simulink model "Test_FourMotor_PID_Ave"  (R2025a)
settings: Solver=ode4  StartTime=0.0  StopTime=2  FixedStep=60e-6  RelTol=1e-3
values from neighbouring files (symbols this model uses):
  Ts = 2e-6    (= 2e-06)    [param.m]
  ts_vec = 60e-6    (= 6e-05)    [param.m]
undefined symbols (not defined in the file or in its folder): DiscIntNeverNeededParam, gcbh, HEV_Param, Limit, magnitude, motorctrl, RPM, sps_rtmsupport
libraries: fl_lib x39, spsCurrentMeasurementLib x26, spsIdealSwitchLib x24, nesl_utility x22, spsVoltageMeasurementLib x21, simulink_extras x13, spsControlledCurrentSourceLib x12, spsControlledVoltageSourceLib x9, slpidlib x7, simulink x6, Uav_Electrical_lib x5, spsSeriesRLCBranchLib x4
(part 4 of 5)

== system Test_FourMotor_PID_Ave/Detailed/Synchronous Motor & Drive1/Three-phase Inverter/Id computation ==
  m : Inport
  Vdc : Inport  Port=2
  Demux : Subsystem
  Demux1 : Subsystem
  Gain : Gain  Gain=Ron
  Math Function : Math  Operator=magnitude^2  SignedPower=on
  Math Function1 : Math  Operator=magnitude^2  SignedPower=on
  Math Function2 : Math  Operator=magnitude^2  SignedPower=on
  Product1 : Product  Inputs=*/  SaturateOnIntegerOverflow=on  OutDataTypeStr=Inherit: Same as first input
  Sum1 : Sum  Inputs=+++  SaturateOnIntegerOverflow=on
  Sum2 : Sum  Inputs=|++  SaturateOnIntegerOverflow=on
  Sum3 : Sum  SaturateOnIntegerOverflow=on
  Unit Delay1 : UnitDelay  SampleTime=Ts  HasFrameUpgradeWarning=on
  Unit Delay4 : UnitDelay  InitialCondition=1  SampleTime=Ts  HasFrameUpgradeWarning=on
  Vac x Ia : Product  SaturateOnIntegerOverflow=on  OutDataTypeStr=Inherit: Same as first input
  Vbc x Ib : Product  SaturateOnIntegerOverflow=on  OutDataTypeStr=Inherit: Same as first input
  Zero avoider : Saturate  UpperLimit=inf  LowerLimit=1
  Id : Outport  VectorParamsAs1DForOutWhenUnconnected=off
  wires:
  Sum2/1 -> Unit Delay1/1
  Sum3/1 -> Sum2/1
  Sum1/1 -> Gain/1
  Math Function2/1 -> Sum1/3
  Math Function/1 -> Sum1/1
  Math Function1/1 -> Sum1/2
  Demux1/3(Ic) -> Math Function2/1
  Demux1/2(Ib) -> Math Function1/1
  Demux1/1(Ia) -> Math Function/1
  Unit Delay4/1 -> Zero avoider/1
  Unit Delay1/1 -> Product1/1
  m/1 -> Demux1/1(m), Demux/1(m)
  Vac x Ia/1 -> Sum3/1
  Vbc x Ib/1 -> Sum3/2
  Vdc/1 -> Unit Delay4/1
  Demux/1(Vac) -> Vac x Ia/1
  Demux/2(Ia) -> Vac x Ia/2
  Demux/4(Ib) -> Vbc x Ib/2
  Demux/3(Vbc) -> Vbc x Ib/1
  Gain/1 -> Sum2/2
  Product1/1 -> Id/1
  Zero avoider/1 -> Product1/2

== system Test_FourMotor_PID_Ave/Detailed/Synchronous Motor & Drive1/Three-phase Inverter/Limit detection ==
  note: Limit = 1 saturation mode (voltage mode)
      | Limit = 0 normal mode (current mode)
  note: Low pass filter
  note: Low pass filter
  Vcc : Inport
  ctrl : Inport  Port=2
  Bus Selector1 : BusSelector  OutputSignals=m.Stator current is_d (A),m.Stator current is_q (A),m.Rotor speed wm (rad/s)  OutputAsBus=on
  Discrete Transfer Fcn1 : DiscreteTransferFcn  Numerator=[1-exp(-Ts*Fcs*2*pi)]  Denominator=[1 -exp(-Ts*Fcs*2*pi)]  SampleTime=Ts
  Discrete Transfer Fcn3 : DiscreteTransferFcn  Numerator=[1-exp(-Ts*Fcs*2*pi)]  Denominator=[1 -exp(-Ts*Fcs*2*pi)]  SampleTime=Ts
  Gain1 : Gain  Gain=0.9  SaturateOnIntegerOverflow=on  OutDataTypeStr=Inherit: Same as input  ParamDataTypeStr=Inherit: Same as input
  "Internal Vcc " : Fcn  Expr=pi/2*sqrt((Resistance*u(1)-Lq*p*u(3)*u(2))^2+(Resistance*u(2)+Ld*p*u(3)*u(1)+Flux*p*u(3))^2)
  Relational Operator : RelationalOperator  Operator=>  OutDataTypeStr=boolean  InputSameDT=off
  Relational Operator2 : RelationalOperator  Operator=<  OutDataTypeStr=boolean  InputSameDT=off
  S-R Flip-Flop : simulink_extras/Flip Flops/S-R Flip-Flop  initial_condition=0
  Terminator : Terminator
  Limit : Outport  VectorParamsAs1DForOutWhenUnconnected=off
  wires:
  Vcc/1 -> Discrete Transfer Fcn3/1
  Relational Operator/1 -> S-R Flip-Flop/1
  Relational Operator2/1 -> S-R Flip-Flop/2
  S-R Flip-Flop/1 -> Limit/1
  ctrl/1 -> Bus Selector1/1
  Bus Selector1/1 -> "Internal Vcc "/1
  "Internal Vcc "/1 -> Discrete Transfer Fcn1/1
  Discrete Transfer Fcn1/1 -> Relational Operator/1, Relational Operator2/1
  Gain1/1 -> Relational Operator2/2
  Discrete Transfer Fcn3/1 -> Gain1/1, Relational Operator/2
  S-R Flip-Flop/2 -> Terminator/1

== system Test_FourMotor_PID_Ave/Detailed/Synchronous Motor & Drive1/Three-phase Inverter/Output Resistance correction ==
  note: Vabc
  ctrl : Inport
  1/R : Gain  Gain=1/(100*Resistance)  SaturateOnIntegerOverflow=on  OutDataTypeStr=Inherit: Same as input  ParamDataTypeStr=Inherit: Same as input
  Bus Selector1 : BusSelector  OutputSignals=m.Stator voltage Vs_d (V),m.Stator voltage Vs_q (V),m.Rotor angle thetam (rad)
  Constant : Constant  Value=0
  Discrete Transfer Fcn1 : DiscreteTransferFcn  Numerator=[1-exp(-Ts/.001)]  Denominator=[1 -exp(-Ts/.001)]  SampleTime=Ts
  Discrete Transfer Fcn2 : DiscreteTransferFcn  Numerator=[1-exp(-Ts/.001)]  Denominator=[1 -exp(-Ts/.001)]  SampleTime=Ts
  Fcn : Fcn  Expr=sin(u)
  Fcn1 : Fcn  Expr=cos(u)
  Mux4 : Mux  Inputs=3
  Mux5 : Mux  Inputs=2
  dq0_to_abc Transformation : powerlib_extras/Measurements/dq0_to_abc Transformation
  poles : Gain  Gain=p  SaturateOnIntegerOverflow=on  OutDataTypeStr=Inherit: Same as input  ParamDataTypeStr=Inherit: Same as input
  "Iabc_r " : Outport  VectorParamsAs1DForOutWhenUnconnected=off
  wires:
  1/R/1 -> "Iabc_r "/1
  Bus Selector1/2 -> Discrete Transfer Fcn2/1  "<Stator voltage Vs_q (V)>"
  Bus Selector1/1 -> Discrete Transfer Fcn1/1  "<Stator voltage Vs_d (V)>"
  ctrl/1 -> Bus Selector1/1
  Mux4/1 -> dq0_to_abc Transformation/1
  Fcn/1 -> Mux5/1
  Fcn1/1 -> Mux5/2
  Mux5/1 -> dq0_to_abc Transformation/2
  Constant/1 -> Mux4/3
  dq0_to_abc Transformation/1 -> 1/R/1
  Discrete Transfer Fcn2/1 -> Mux4/2
  Discrete Transfer Fcn1/1 -> Mux4/1
  Bus Selector1/3 -> poles/1  "<Rotor angle thetam (rad)>"
  poles/1 -> Fcn/1, Fcn1/1

== system Test_FourMotor_PID_Ave/Detailed/Synchronous Motor & Drive1/VECT Controller/Current Regulator1 ==
  Iabc* : Inport
  Iabc : Inport  Port=2
  BusCreator : BusCreator  Inputs=6
  Data Type Conversion{,1..5} (6 alike) : DataTypeConversion
  Demux1 : Demux  Outputs=3
      settings: DisplayOption=none
  Demux2 : Demux  Outputs=3
      settings: DisplayOption=none
  Logical Operator : Logic  Operator=NOT
  Logical Operator1 : Logic  Operator=NOT
  Logical Operator2 : Logic  Operator=NOT
  Relay : Relay  OnSwitchValue=h/2  OffSwitchValue=-h/2
  Relay1 : Relay  OnSwitchValue=h/2  OffSwitchValue=-h/2
  Relay2 : Relay  OnSwitchValue=h/2  OffSwitchValue=-h/2
  Sum : Sum  Inputs=-+  InputSameDT=on  SaturateOnIntegerOverflow=on  OutDataTypeStr=Inherit: Same as first input
  Sum1 : Sum  Inputs=-+  InputSameDT=on  SaturateOnIntegerOverflow=on  OutDataTypeStr=Inherit: Same as first input
  Sum2 : Sum  Inputs=-+  InputSameDT=on  SaturateOnIntegerOverflow=on  OutDataTypeStr=Inherit: Same as first input
  Pulses : Outport  InitialOutput=0  VectorParamsAs1DForOutWhenUnconnected=off
  wires:
  Data Type Conversion5/1 -> BusCreator/6
  Data Type Conversion4/1 -> Logical Operator2/1
  Data Type Conversion3/1 -> BusCreator/4
  Data Type Conversion2/1 -> Logical Operator1/1
  Data Type Conversion1/1 -> BusCreator/2
  Data Type Conversion/1 -> Logical Operator/1
  Sum/1 -> Relay/1
  Sum1/1 -> Relay1/1
  Demux1/1 -> Sum/1
  Demux1/2 -> Sum1/1
  BusCreator/1 -> Pulses/1
  Iabc/1 -> Demux1/1
  Sum2/1 -> Relay2/1
  Demux1/3 -> Sum2/1
  Demux2/3 -> Sum2/2
  Demux2/2 -> Sum1/2
  Demux2/1 -> Sum/2
  Iabc*/1 -> Demux2/1
  Relay/1 -> Data Type Conversion/1, BusCreator/1
  Relay1/1 -> Data Type Conversion2/1, BusCreator/3
  Relay2/1 -> Data Type Conversion4/1, BusCreator/5
  Logical Operator/1 -> Data Type Conversion1/1
  Logical Operator1/1 -> Data Type Conversion3/1
  Logical Operator2/1 -> Data Type Conversion5/1

== system Test_FourMotor_PID_Ave/Detailed/Synchronous Motor & Drive1/VECT Controller/DQ-ABC ==
  "Iq* " : Inport
  "Id* " : Inport  Port=2
  Teta : Inport  Port=3
  Fcn : Fcn  Expr=sin(u)
  Fcn1 : Fcn  Expr=cos(u)
  Gain2 : Gain  SaturateOnIntegerOverflow=on  OutDataTypeStr=Inherit: Same as input  ParamDataTypeStr=Inherit: Same as input
  Gain3 : Gain  SaturateOnIntegerOverflow=on  OutDataTypeStr=Inherit: Same as input  ParamDataTypeStr=Inherit: Same as input
  Gain4 : Gain  SaturateOnIntegerOverflow=on  OutDataTypeStr=Inherit: Same as input  ParamDataTypeStr=Inherit: Same as input
  Mux : Mux
  Mux2 : Mux  Inputs=3
  ia : Fcn  Expr=-u[3]*u[2] + u[4]*u[1]
  ib : Fcn  Expr=(-u[1]+1.7320508*u[2])*u[4]*0.5+(u[2]+1.7320508*u[1])*u[3]*0.5
  ic : Sum  Inputs=--  InputSameDT=on  SaturateOnIntegerOverflow=on  OutDataTypeStr=Inherit: Same as first input
  Iabc* : Outport  InitialOutput=0  VectorParamsAs1DForOutWhenUnconnected=off
  wires:
  ib/1 -> ic/1, Gain3/1
  ia/1 -> ic/2, Gain2/1
  Gain2/1 -> Mux2/1
  Gain4/1 -> Mux2/3
  ic/1 -> Gain4/1
  Gain3/1 -> Mux2/2
  "Iq* "/1 -> Mux/4
  "Id* "/1 -> Mux/3
  Teta/1 -> Fcn/1, Fcn1/1
  Mux/1 -> ia/1, ib/1
  Mux2/1 -> Iabc*/1
  Fcn1/1 -> Mux/1
  Fcn/1 -> Mux/2

== system Test_FourMotor_PID_Ave/Detailed/Synchronous Motor & Drive2/Three-phase Inverter/Activation Switches ==
  gate : Inport
  Ideal Switch1 : spsIdealSwitchLib/Ideal Switch  Ron=2*Ron  Lon=0  IC=1  Rs=1e6  Cs=inf  Measurements=off
  Ideal Switch2 : spsIdealSwitchLib/Ideal Switch  Ron=2*Ron  Lon=0  IC=1  Rs=1e6  Cs=inf  Measurements=off
  Ideal Switch3 : spsIdealSwitchLib/Ideal Switch  Ron=2*Ron  Lon=0  IC=1  Rs=1e6  Cs=inf  Measurements=off
  Ideal Switch4 : spsIdealSwitchLib/Ideal Switch  Ron=2*Ron  Lon=0  IC=0  Rs=1e6  Cs=inf  Measurements=off
  Ideal Switch5 : spsIdealSwitchLib/Ideal Switch  Ron=2*Ron  Lon=0  IC=0  Rs=1e6  Cs=inf  Measurements=off
  Ideal Switch6 : spsIdealSwitchLib/Ideal Switch  Ron=2*Ron  Lon=0  IC=0  Rs=1e6  Cs=inf  Measurements=off
  Logical Operator : Logic  Operator=NOT  AllPortsSameDT=off  OutDataTypeStr=boolean
  A1 : PMIOPort  Side=Left
  a : PMIOPort  Port=2  Side=Right
  B1 : PMIOPort  Port=3  Side=Left
  b : PMIOPort  Port=4  Side=Right
  C1 : PMIOPort  Port=5  Side=Left
  c : PMIOPort  Port=6  Side=Right
  A2 : PMIOPort  Port=7  Side=Left
  B2 : PMIOPort  Port=8  Side=Left
  C2 : PMIOPort  Port=9  Side=Left
  wires:
  gate/1 -> Ideal Switch1/1, Ideal Switch2/1, Ideal Switch3/1, Logical Operator/1
  Logical Operator/1 -> Ideal Switch4/1, Ideal Switch5/1, Ideal Switch6/1
  connections:
  A1/RConn1 -- Ideal Switch1/LConn1
  Ideal Switch1/RConn1 -- a/RConn1 -- Ideal Switch4/RConn1
  B1/RConn1 -- Ideal Switch2/LConn1
  Ideal Switch2/RConn1 -- Ideal Switch5/RConn1 -- b/RConn1
  C1/RConn1 -- Ideal Switch3/LConn1
  Ideal Switch3/RConn1 -- Ideal Switch6/RConn1 -- c/RConn1
  A2/RConn1 -- Ideal Switch4/LConn1
  B2/RConn1 -- Ideal Switch5/LConn1
  C2/RConn1 -- Ideal Switch6/LConn1

== system Test_FourMotor_PID_Ave/Detailed/Synchronous Motor & Drive2/Three-phase Inverter/Id computation ==
  m : Inport
  Vdc : Inport  Port=2
  Demux : Subsystem
  Demux1 : Subsystem
  Gain : Gain  Gain=Ron
  Math Function : Math  Operator=magnitude^2  SignedPower=on
  Math Function1 : Math  Operator=magnitude^2  SignedPower=on
  Math Function2 : Math  Operator=magnitude^2  SignedPower=on
  Product1 : Product  Inputs=*/  SaturateOnIntegerOverflow=on  OutDataTypeStr=Inherit: Same as first input
  Sum1 : Sum  Inputs=+++  SaturateOnIntegerOverflow=on
  Sum2 : Sum  Inputs=|++  SaturateOnIntegerOverflow=on
  Sum3 : Sum  SaturateOnIntegerOverflow=on
  Unit Delay1 : UnitDelay  SampleTime=Ts  HasFrameUpgradeWarning=on
  Unit Delay4 : UnitDelay  InitialCondition=1  SampleTime=Ts  HasFrameUpgradeWarning=on
  Vac x Ia : Product  SaturateOnIntegerOverflow=on  OutDataTypeStr=Inherit: Same as first input
  Vbc x Ib : Product  SaturateOnIntegerOverflow=on  OutDataTypeStr=Inherit: Same as first input
  Zero avoider : Saturate  UpperLimit=inf  LowerLimit=1
  Id : Outport  VectorParamsAs1DForOutWhenUnconnected=off
  wires:
  Sum2/1 -> Unit Delay1/1
  Sum3/1 -> Sum2/1
  Sum1/1 -> Gain/1
  Math Function2/1 -> Sum1/3
  Math Function/1 -> Sum1/1
  Math Function1/1 -> Sum1/2
  Demux1/3(Ic) -> Math Function2/1
  Demux1/2(Ib) -> Math Function1/1
  Demux1/1(Ia) -> Math Function/1
  Unit Delay4/1 -> Zero avoider/1
  Unit Delay1/1 -> Product1/1
  m/1 -> Demux1/1(m), Demux/1(m)
  Vac x Ia/1 -> Sum3/1
  Vbc x Ib/1 -> Sum3/2
  Vdc/1 -> Unit Delay4/1
  Demux/1(Vac) -> Vac x Ia/1
  Demux/2(Ia) -> Vac x Ia/2
  Demux/4(Ib) -> Vbc x Ib/2
  Demux/3(Vbc) -> Vbc x Ib/1
  Gain/1 -> Sum2/2
  Product1/1 -> Id/1
  Zero avoider/1 -> Product1/2

== system Test_FourMotor_PID_Ave/Detailed/Synchronous Motor & Drive2/Three-phase Inverter/Limit detection ==
  note: Limit = 1 saturation mode (voltage mode)
      | Limit = 0 normal mode (current mode)
  note: Low pass filter
  note: Low pass filter
  Vcc : Inport
  ctrl : Inport  Port=2
  Bus Selector1 : BusSelector  OutputSignals=m.Stator current is_d (A),m.Stator current is_q (A),m.Rotor speed wm (rad/s)  OutputAsBus=on
  Discrete Transfer Fcn1 : DiscreteTransferFcn  Numerator=[1-exp(-Ts*Fcs*2*pi)]  Denominator=[1 -exp(-Ts*Fcs*2*pi)]  SampleTime=Ts
  Discrete Transfer Fcn3 : DiscreteTransferFcn  Numerator=[1-exp(-Ts*Fcs*2*pi)]  Denominator=[1 -exp(-Ts*Fcs*2*pi)]  SampleTime=Ts
  Gain1 : Gain  Gain=0.9  SaturateOnIntegerOverflow=on  OutDataTypeStr=Inherit: Same as input  ParamDataTypeStr=Inherit: Same as input
  "Internal Vcc " : Fcn  Expr=pi/2*sqrt((Resistance*u(1)-Lq*p*u(3)*u(2))^2+(Resistance*u(2)+Ld*p*u(3)*u(1)+Flux*p*u(3))^2)
  Relational Operator : RelationalOperator  Operator=>  OutDataTypeStr=boolean  InputSameDT=off
  Relational Operator2 : RelationalOperator  Operator=<  OutDataTypeStr=boolean  InputSameDT=off
  S-R Flip-Flop : simulink_extras/Flip Flops/S-R Flip-Flop  initial_condition=0
  Terminator : Terminator
  Limit : Outport  VectorParamsAs1DForOutWhenUnconnected=off
  wires:
  Vcc/1 -> Discrete Transfer Fcn3/1
  Relational Operator/1 -> S-R Flip-Flop/1
  Relational Operator2/1 -> S-R Flip-Flop/2
  S-R Flip-Flop/1 -> Limit/1
  ctrl/1 -> Bus Selector1/1
  Bus Selector1/1 -> "Internal Vcc "/1
  "Internal Vcc "/1 -> Discrete Transfer Fcn1/1
  Discrete Transfer Fcn1/1 -> Relational Operator/1, Relational Operator2/1
  Gain1/1 -> Relational Operator2/2
  Discrete Transfer Fcn3/1 -> Gain1/1, Relational Operator/2
  S-R Flip-Flop/2 -> Terminator/1

== system Test_FourMotor_PID_Ave/Detailed/Synchronous Motor & Drive2/Three-phase Inverter/Output Resistance correction ==
  note: Vabc
  ctrl : Inport
  1/R : Gain  Gain=1/(100*Resistance)  SaturateOnIntegerOverflow=on  OutDataTypeStr=Inherit: Same as input  ParamDataTypeStr=Inherit: Same as input
  Bus Selector1 : BusSelector  OutputSignals=m.Stator voltage Vs_d (V),m.Stator voltage Vs_q (V),m.Rotor angle thetam (rad)
  Constant : Constant  Value=0
  Discrete Transfer Fcn1 : DiscreteTransferFcn  Numerator=[1-exp(-Ts/.001)]  Denominator=[1 -exp(-Ts/.001)]  SampleTime=Ts
  Discrete Transfer Fcn2 : DiscreteTransferFcn  Numerator=[1-exp(-Ts/.001)]  Denominator=[1 -exp(-Ts/.001)]  SampleTime=Ts
  Fcn : Fcn  Expr=sin(u)
  Fcn1 : Fcn  Expr=cos(u)
  Mux4 : Mux  Inputs=3
  Mux5 : Mux  Inputs=2
  dq0_to_abc Transformation : powerlib_extras/Measurements/dq0_to_abc Transformation
  poles : Gain  Gain=p  SaturateOnIntegerOverflow=on  OutDataTypeStr=Inherit: Same as input  ParamDataTypeStr=Inherit: Same as input
  "Iabc_r " : Outport  VectorParamsAs1DForOutWhenUnconnected=off
  wires:
  1/R/1 -> "Iabc_r "/1
  Bus Selector1/2 -> Discrete Transfer Fcn2/1  "<Stator voltage Vs_q (V)>"
  Bus Selector1/1 -> Discrete Transfer Fcn1/1  "<Stator voltage Vs_d (V)>"
  ctrl/1 -> Bus Selector1/1
  Mux4/1 -> dq0_to_abc Transformation/1
  Fcn/1 -> Mux5/1
  Fcn1/1 -> Mux5/2
  Mux5/1 -> dq0_to_abc Transformation/2
  Constant/1 -> Mux4/3
  dq0_to_abc Transformation/1 -> 1/R/1
  Discrete Transfer Fcn2/1 -> Mux4/2
  Discrete Transfer Fcn1/1 -> Mux4/1
  Bus Selector1/3 -> poles/1  "<Rotor angle thetam (rad)>"
  poles/1 -> Fcn/1, Fcn1/1

== system Test_FourMotor_PID_Ave/Detailed/Synchronous Motor & Drive2/VECT controller/Current Regulator ==
  Iabc* : Inport
  Iabc : Inport  Port=2
  Demux1 : Demux  Outputs=3
      settings: DisplayOption=none
  Demux2 : Demux  Outputs=3
      settings: DisplayOption=none
  Mux1 : Mux  Inputs=2
  Relay : Relay  OnSwitchValue=0  OffSwitchValue=0
  Relay1 : Relay  OnSwitchValue=0  OffSwitchValue=0
  Relay2 : Relay  OnSwitchValue=0  OffSwitchValue=0
  Sum : Sum  Inputs=-+  InputSameDT=on  SaturateOnIntegerOverflow=on  OutDataTypeStr=Inherit: Same as first input
  Sum1 : Sum  Inputs=-+  InputSameDT=on  SaturateOnIntegerOverflow=on  OutDataTypeStr=Inherit: Same as first input
  Sum2 : Sum  Inputs=-+  InputSameDT=on  SaturateOnIntegerOverflow=on  OutDataTypeStr=Inherit: Same as first input
  Sum3 : Sum  Inputs=+-
  Sum4 : Sum  Inputs=+-
  Pulses : Outport  InitialOutput=0  VectorParamsAs1DForOutWhenUnconnected=off
  wires:
  Sum/1 -> Relay/1
  Sum1/1 -> Relay1/1
  Demux1/1 -> Sum/1
  Demux1/2 -> Sum1/1
  Mux1/1 -> Pulses/1
  Iabc/1 -> Demux1/1
  Sum2/1 -> Relay2/1
  Demux1/3 -> Sum2/1
  Demux2/3 -> Sum2/2
  Demux2/2 -> Sum1/2
  Demux2/1 -> Sum/2
  Iabc*/1 -> Demux2/1
  Relay/1 -> Sum3/1
  Relay1/1 -> Sum3/2, Sum4/1
  Relay2/1 -> Sum4/2
  Sum3/1 -> Mux1/1
  Sum4/1 -> Mux1/2

== system Test_FourMotor_PID_Ave/Detailed/Synchronous Motor & Drive2/VECT controller/DQ-ABC ==
  "Iq* " : Inport
  "Id* " : Inport  Port=2
  Teta : Inport  Port=3
  Fcn : Fcn  Expr=sin(u)
  Fcn1 : Fcn  Expr=cos(u)
  Gain2 : Gain  SaturateOnIntegerOverflow=on  OutDataTypeStr=Inherit: Same as input  ParamDataTypeStr=Inherit: Same as input
  Gain3 : Gain  SaturateOnIntegerOverflow=on  OutDataTypeStr=Inherit: Same as input  ParamDataTypeStr=Inherit: Same as input
  Gain4 : Gain  SaturateOnIntegerOverflow=on  OutDataTypeStr=Inherit: Same as input  ParamDataTypeStr=Inherit: Same as input
  Mux : Mux
  Mux2 : Mux  Inputs=3
  ia : Fcn  Expr=-u[3]*u[2] + u[4]*u[1]
  ib : Fcn  Expr=(-u[1]+1.7320508*u[2])*u[4]*0.5+(u[2]+1.7320508*u[1])*u[3]*0.5
  ic : Sum  Inputs=--  InputSameDT=on  SaturateOnIntegerOverflow=on  OutDataTypeStr=Inherit: Same as first input
  Iabc* : Outport  InitialOutput=0  VectorParamsAs1DForOutWhenUnconnected=off
  wires:
  Fcn/1 -> Mux/2
  Fcn1/1 -> Mux/1
  Mux2/1 -> Iabc*/1
  Mux/1 -> ib/1, ia/1
  Teta/1 -> Fcn1/1, Fcn/1
  "Id* "/1 -> Mux/3
  "Iq* "/1 -> Mux/4
  Gain3/1 -> Mux2/2
  ic/1 -> Gain4/1
  Gain4/1 -> Mux2/3
  Gain2/1 -> Mux2/1
  ia/1 -> Gain2/1, ic/2
  ib/1 -> Gain3/1, ic/1

== system Test_FourMotor_PID_Ave/Detailed/Synchronous Motor & Drive2/VECT controller/Zero crossing detector ==
  En : Inport
  Iabc* : Inport  Port=2
  D Latch : simulink_extras/Flip Flops/D Latch
  D Latch1 : simulink_extras/Flip Flops/D Latch
  D Latch2 : simulink_extras/Flip Flops/D Latch
  Data Type Conversion : DataTypeConversion  SaturateOnIntegerOverflow=off  RndMeth=Floor
  Data Type Conversion2 : DataTypeConversion  SaturateOnIntegerOverflow=off  RndMeth=Floor
  Demux : Demux  Outputs=3
  Hit Crossing : HitCross
  Mux : Mux  Inputs=3
  Terminator : Terminator
  Terminator1 : Terminator
  Terminator2 : Terminator
  Enable : Outport  VectorParamsAs1DForOutWhenUnconnected=off
  wires:
  Data Type Conversion/1 -> D Latch/1, D Latch1/1, D Latch2/1
  Hit Crossing/1 -> Demux/1
  Demux/2 -> D Latch1/2
  Demux/3 -> D Latch2/2
  D Latch/1 -> Mux/1
  D Latch1/1 -> Mux/2
  D Latch2/1 -> Mux/3
  Mux/1 -> Data Type Conversion2/1
  Demux/1 -> D Latch/2
  En/1 -> Data Type Conversion/1
  Iabc*/1 -> Hit Crossing/1
  Data Type Conversion2/1 -> Enable/1
  D Latch/2 -> Terminator/1
  D Latch1/2 -> Terminator1/1
  D Latch2/2 -> Terminator2/1

== system Test_FourMotor_PID_Ave/Detailed/Synchronous Motor & Drive3/Three-phase Inverter/Activation Switches ==
  gate : Inport
  Ideal Switch1 : spsIdealSwitchLib/Ideal Switch  Ron=2*Ron  Lon=0  IC=1  Rs=1e6  Cs=inf  Measurements=off
  Ideal Switch2 : spsIdealSwitchLib/Ideal Switch  Ron=2*Ron  Lon=0  IC=1  Rs=1e6  Cs=inf  Measurements=off
  Ideal Switch3 : spsIdealSwitchLib/Ideal Switch  Ron=2*Ron  Lon=0  IC=1  Rs=1e6  Cs=inf  Measurements=off
  Ideal Switch4 : spsIdealSwitchLib/Ideal Switch  Ron=2*Ron  Lon=0  IC=0  Rs=1e6  Cs=inf  Measurements=off
  Ideal Switch5 : spsIdealSwitchLib/Ideal Switch  Ron=2*Ron  Lon=0  IC=0  Rs=1e6  Cs=inf  Measurements=off
  Ideal Switch6 : spsIdealSwitchLib/Ideal Switch  Ron=2*Ron  Lon=0  IC=0  Rs=1e6  Cs=inf  Measurements=off
  Logical Operator : Logic  Operator=NOT  AllPortsSameDT=off  OutDataTypeStr=boolean
  A1 : PMIOPort  Side=Left
  a : PMIOPort  Port=2  Side=Right
  B1 : PMIOPort  Port=3  Side=Left
  b : PMIOPort  Port=4  Side=Right
  C1 : PMIOPort  Port=5  Side=Left
  c : PMIOPort  Port=6  Side=Right
  A2 : PMIOPort  Port=7  Side=Left
  B2 : PMIOPort  Port=8  Side=Left
  C2 : PMIOPort  Port=9  Side=Left
  wires:
  gate/1 -> Ideal Switch1/1, Ideal Switch2/1, Ideal Switch3/1, Logical Operator/1
  Logical Operator/1 -> Ideal Switch4/1, Ideal Switch5/1, Ideal Switch6/1
  connections:
  A1/RConn1 -- Ideal Switch1/LConn1
  Ideal Switch1/RConn1 -- a/RConn1 -- Ideal Switch4/RConn1
  B1/RConn1 -- Ideal Switch2/LConn1
  Ideal Switch2/RConn1 -- Ideal Switch5/RConn1 -- b/RConn1
  C1/RConn1 -- Ideal Switch3/LConn1
  Ideal Switch3/RConn1 -- Ideal Switch6/RConn1 -- c/RConn1
  A2/RConn1 -- Ideal Switch4/LConn1
  B2/RConn1 -- Ideal Switch5/LConn1
  C2/RConn1 -- Ideal Switch6/LConn1

== system Test_FourMotor_PID_Ave/Detailed/Synchronous Motor & Drive3/Three-phase Inverter/Id computation ==
  m : Inport
  Vdc : Inport  Port=2
  Demux : Subsystem
  Demux1 : Subsystem
  Gain : Gain  Gain=Ron
  Math Function : Math  Operator=magnitude^2  SignedPower=on
  Math Function1 : Math  Operator=magnitude^2  SignedPower=on
  Math Function2 : Math  Operator=magnitude^2  SignedPower=on
  Product1 : Product  Inputs=*/  SaturateOnIntegerOverflow=on  OutDataTypeStr=Inherit: Same as first input
  Sum1 : Sum  Inputs=+++  SaturateOnIntegerOverflow=on
  Sum2 : Sum  Inputs=|++  SaturateOnIntegerOverflow=on
  Sum3 : Sum  SaturateOnIntegerOverflow=on
  Unit Delay1 : UnitDelay  SampleTime=Ts  HasFrameUpgradeWarning=on
  Unit Delay4 : UnitDelay  InitialCondition=1  SampleTime=Ts  HasFrameUpgradeWarning=on
  Vac x Ia : Product  SaturateOnIntegerOverflow=on  OutDataTypeStr=Inherit: Same as first input
  Vbc x Ib : Product  SaturateOnIntegerOverflow=on  OutDataTypeStr=Inherit: Same as first input
  Zero avoider : Saturate  UpperLimit=inf  LowerLimit=1
  Id : Outport  VectorParamsAs1DForOutWhenUnconnected=off
  wires:
  Sum2/1 -> Unit Delay1/1
  Sum3/1 -> Sum2/1
  Sum1/1 -> Gain/1
  Math Function2/1 -> Sum1/3
  Math Function/1 -> Sum1/1
  Math Function1/1 -> Sum1/2
  Demux1/3(Ic) -> Math Function2/1
  Demux1/2(Ib) -> Math Function1/1
  Demux1/1(Ia) -> Math Function/1
  Unit Delay4/1 -> Zero avoider/1
  Unit Delay1/1 -> Product1/1
  m/1 -> Demux1/1(m), Demux/1(m)
  Vac x Ia/1 -> Sum3/1
  Vbc x Ib/1 -> Sum3/2
  Vdc/1 -> Unit Delay4/1
  Demux/1(Vac) -> Vac x Ia/1
  Demux/2(Ia) -> Vac x Ia/2
  Demux/4(Ib) -> Vbc x Ib/2
  Demux/3(Vbc) -> Vbc x Ib/1
  Gain/1 -> Sum2/2
  Product1/1 -> Id/1
  Zero avoider/1 -> Product1/2

== system Test_FourMotor_PID_Ave/Detailed/Synchronous Motor & Drive3/Three-phase Inverter/Limit detection ==
  note: Limit = 1 saturation mode (voltage mode)
      | Limit = 0 normal mode (current mode)
  note: Low pass filter
  note: Low pass filter
  Vcc : Inport
  ctrl : Inport  Port=2
  Bus Selector1 : BusSelector  OutputSignals=m.Stator current is_d (A),m.Stator current is_q (A),m.Rotor speed wm (rad/s)  OutputAsBus=on
  Discrete Transfer Fcn1 : DiscreteTransferFcn  Numerator=[1-exp(-Ts*Fcs*2*pi)]  Denominator=[1 -exp(-Ts*Fcs*2*pi)]  SampleTime=Ts
  Discrete Transfer Fcn3 : DiscreteTransferFcn  Numerator=[1-exp(-Ts*Fcs*2*pi)]  Denominator=[1 -exp(-Ts*Fcs*2*pi)]  SampleTime=Ts
  Gain1 : Gain  Gain=0.9  SaturateOnIntegerOverflow=on  OutDataTypeStr=Inherit: Same as input  ParamDataTypeStr=Inherit: Same as input
  "Internal Vcc " : Fcn  Expr=pi/2*sqrt((Resistance*u(1)-Lq*p*u(3)*u(2))^2+(Resistance*u(2)+Ld*p*u(3)*u(1)+Flux*p*u(3))^2)
  Relational Operator : RelationalOperator  Operator=>  OutDataTypeStr=boolean  InputSameDT=off
  Relational Operator2 : RelationalOperator  Operator=<  OutDataTypeStr=boolean  InputSameDT=off
  S-R Flip-Flop : simulink_extras/Flip Flops/S-R Flip-Flop  initial_condition=0
  Terminator : Terminator
  Limit : Outport  VectorParamsAs1DForOutWhenUnconnected=off
  wires:
  Vcc/1 -> Discrete Transfer Fcn3/1
  Relational Operator/1 -> S-R Flip-Flop/1
  Relational Operator2/1 -> S-R Flip-Flop/2
  S-R Flip-Flop/1 -> Limit/1
  ctrl/1 -> Bus Selector1/1
  Bus Selector1/1 -> "Internal Vcc "/1
  "Internal Vcc "/1 -> Discrete Transfer Fcn1/1
  Discrete Transfer Fcn1/1 -> Relational Operator/1, Relational Operator2/1
  Gain1/1 -> Relational Operator2/2
  Discrete Transfer Fcn3/1 -> Gain1/1, Relational Operator/2
  S-R Flip-Flop/2 -> Terminator/1

== system Test_FourMotor_PID_Ave/Detailed/Synchronous Motor & Drive3/Three-phase Inverter/Output Resistance correction ==
  note: Vabc
  ctrl : Inport
  1/R : Gain  Gain=1/(100*Resistance)  SaturateOnIntegerOverflow=on  OutDataTypeStr=Inherit: Same as input  ParamDataTypeStr=Inherit: Same as input
  Bus Selector1 : BusSelector  OutputSignals=m.Stator voltage Vs_d (V),m.Stator voltage Vs_q (V),m.Rotor angle thetam (rad)
  Constant : Constant  Value=0
  Discrete Transfer Fcn1 : DiscreteTransferFcn  Numerator=[1-exp(-Ts/.001)]  Denominator=[1 -exp(-Ts/.001)]  SampleTime=Ts
  Discrete Transfer Fcn2 : DiscreteTransferFcn  Numerator=[1-exp(-Ts/.001)]  Denominator=[1 -exp(-Ts/.001)]  SampleTime=Ts
  Fcn : Fcn  Expr=sin(u)
  Fcn1 : Fcn  Expr=cos(u)
  Mux4 : Mux  Inputs=3
  Mux5 : Mux  Inputs=2
  dq0_to_abc Transformation : powerlib_extras/Measurements/dq0_to_abc Transformation
  poles : Gain  Gain=p  SaturateOnIntegerOverflow=on  OutDataTypeStr=Inherit: Same as input  ParamDataTypeStr=Inherit: Same as input
  "Iabc_r " : Outport  VectorParamsAs1DForOutWhenUnconnected=off
  wires:
  1/R/1 -> "Iabc_r "/1
  Bus Selector1/2 -> Discrete Transfer Fcn2/1  "<Stator voltage Vs_q (V)>"
  Bus Selector1/1 -> Discrete Transfer Fcn1/1  "<Stator voltage Vs_d (V)>"
  ctrl/1 -> Bus Selector1/1
  Mux4/1 -> dq0_to_abc Transformation/1
  Fcn/1 -> Mux5/1
  Fcn1/1 -> Mux5/2
  Mux5/1 -> dq0_to_abc Transformation/2
  Constant/1 -> Mux4/3
  dq0_to_abc Transformation/1 -> 1/R/1
  Discrete Transfer Fcn2/1 -> Mux4/2
  Discrete Transfer Fcn1/1 -> Mux4/1
  Bus Selector1/3 -> poles/1  "<Rotor angle thetam (rad)>"
  poles/1 -> Fcn/1, Fcn1/1

== system Test_FourMotor_PID_Ave/Detailed/Synchronous Motor & Drive3/VECT controller/Current Regulator ==
  Iabc* : Inport
  Iabc : Inport  Port=2
  Demux1 : Demux  Outputs=3
      settings: DisplayOption=none
  Demux2 : Demux  Outputs=3
      settings: DisplayOption=none
  Mux1 : Mux  Inputs=2
  Relay : Relay  OnSwitchValue=0  OffSwitchValue=0
  Relay1 : Relay  OnSwitchValue=0  OffSwitchValue=0
  Relay2 : Relay  OnSwitchValue=0  OffSwitchValue=0
  Sum : Sum  Inputs=-+  InputSameDT=on  SaturateOnIntegerOverflow=on  OutDataTypeStr=Inherit: Same as first input
  Sum1 : Sum  Inputs=-+  InputSameDT=on  SaturateOnIntegerOverflow=on  OutDataTypeStr=Inherit: Same as first input
  Sum2 : Sum  Inputs=-+  InputSameDT=on  SaturateOnIntegerOverflow=on  OutDataTypeStr=Inherit: Same as first input
  Sum3 : Sum  Inputs=+-
  Sum4 : Sum  Inputs=+-
  Pulses : Outport  InitialOutput=0  VectorParamsAs1DForOutWhenUnconnected=off
  wires:
  Sum/1 -> Relay/1
  Sum1/1 -> Relay1/1
  Demux1/1 -> Sum/1
  Demux1/2 -> Sum1/1
  Mux1/1 -> Pulses/1
  Iabc/1 -> Demux1/1
  Sum2/1 -> Relay2/1
  Demux1/3 -> Sum2/1
  Demux2/3 -> Sum2/2
  Demux2/2 -> Sum1/2
  Demux2/1 -> Sum/2
  Iabc*/1 -> Demux2/1
  Relay/1 -> Sum3/1
  Relay1/1 -> Sum3/2, Sum4/1
  Relay2/1 -> Sum4/2
  Sum3/1 -> Mux1/1
  Sum4/1 -> Mux1/2

== system Test_FourMotor_PID_Ave/Detailed/Synchronous Motor & Drive3/VECT controller/DQ-ABC ==
  "Iq* " : Inport
  "Id* " : Inport  Port=2
  Teta : Inport  Port=3
  Fcn : Fcn  Expr=sin(u)
  Fcn1 : Fcn  Expr=cos(u)
  Gain2 : Gain  SaturateOnIntegerOverflow=on  OutDataTypeStr=Inherit: Same as input  ParamDataTypeStr=Inherit: Same as input
  Gain3 : Gain  SaturateOnIntegerOverflow=on  OutDataTypeStr=Inherit: Same as input  ParamDataTypeStr=Inherit: Same as input
  Gain4 : Gain  SaturateOnIntegerOverflow=on  OutDataTypeStr=Inherit: Same as input  ParamDataTypeStr=Inherit: Same as input
  Mux : Mux
  Mux2 : Mux  Inputs=3
  ia : Fcn  Expr=-u[3]*u[2] + u[4]*u[1]
  ib : Fcn  Expr=(-u[1]+1.7320508*u[2])*u[4]*0.5+(u[2]+1.7320508*u[1])*u[3]*0.5
  ic : Sum  Inputs=--  InputSameDT=on  SaturateOnIntegerOverflow=on  OutDataTypeStr=Inherit: Same as first input
  Iabc* : Outport  InitialOutput=0  VectorParamsAs1DForOutWhenUnconnected=off
  wires:
  Fcn/1 -> Mux/2
  Fcn1/1 -> Mux/1
  Mux2/1 -> Iabc*/1
  Mux/1 -> ib/1, ia/1
  Teta/1 -> Fcn1/1, Fcn/1
  "Id* "/1 -> Mux/3
  "Iq* "/1 -> Mux/4
  Gain3/1 -> Mux2/2
  ic/1 -> Gain4/1
  Gain4/1 -> Mux2/3
  Gain2/1 -> Mux2/1
  ia/1 -> Gain2/1, ic/2
  ib/1 -> Gain3/1, ic/1

== system Test_FourMotor_PID_Ave/Detailed/Synchronous Motor & Drive3/VECT controller/Zero crossing detector ==
  En : Inport
  Iabc* : Inport  Port=2
  D Latch : simulink_extras/Flip Flops/D Latch
  D Latch1 : simulink_extras/Flip Flops/D Latch
  D Latch2 : simulink_extras/Flip Flops/D Latch
  Data Type Conversion : DataTypeConversion  SaturateOnIntegerOverflow=off  RndMeth=Floor
  Data Type Conversion2 : DataTypeConversion  SaturateOnIntegerOverflow=off  RndMeth=Floor
  Demux : Demux  Outputs=3
  Hit Crossing : HitCross
  Mux : Mux  Inputs=3
  Terminator : Terminator
  Terminator1 : Terminator
  Terminator2 : Terminator
  Enable : Outport  VectorParamsAs1DForOutWhenUnconnected=off
  wires:
  Data Type Conversion/1 -> D Latch/1, D Latch1/1, D Latch2/1
  Hit Crossing/1 -> Demux/1
  Demux/2 -> D Latch1/2
  Demux/3 -> D Latch2/2
  D Latch/1 -> Mux/1
  D Latch1/1 -> Mux/2
  D Latch2/1 -> Mux/3
  Mux/1 -> Data Type Conversion2/1
  Demux/1 -> D Latch/2
  En/1 -> Data Type Conversion/1
  Iabc*/1 -> Hit Crossing/1
  Data Type Conversion2/1 -> Enable/1
  D Latch/2 -> Terminator/1
  D Latch1/2 -> Terminator1/1
  D Latch2/2 -> Terminator2/1

== system Test_FourMotor_PID_Ave/Detailed/Synchronous Motor & Drive4/Three-phase Inverter/Activation Switches ==
  gate : Inport
  Ideal Switch1 : spsIdealSwitchLib/Ideal Switch  Ron=2*Ron  Lon=0  IC=1  Rs=1e6  Cs=inf  Measurements=off
  Ideal Switch2 : spsIdealSwitchLib/Ideal Switch  Ron=2*Ron  Lon=0  IC=1  Rs=1e6  Cs=inf  Measurements=off
  Ideal Switch3 : spsIdealSwitchLib/Ideal Switch  Ron=2*Ron  Lon=0  IC=1  Rs=1e6  Cs=inf  Measurements=off
  Ideal Switch4 : spsIdealSwitchLib/Ideal Switch  Ron=2*Ron  Lon=0  IC=0  Rs=1e6  Cs=inf  Measurements=off
  Ideal Switch5 : spsIdealSwitchLib/Ideal Switch  Ron=2*Ron  Lon=0  IC=0  Rs=1e6  Cs=inf  Measurements=off
  Ideal Switch6 : spsIdealSwitchLib/Ideal Switch  Ron=2*Ron  Lon=0  IC=0  Rs=1e6  Cs=inf  Measurements=off
  Logical Operator : Logic  Operator=NOT  AllPortsSameDT=off  OutDataTypeStr=boolean
  A1 : PMIOPort  Side=Left
  a : PMIOPort  Port=2  Side=Right
  B1 : PMIOPort  Port=3  Side=Left
  b : PMIOPort  Port=4  Side=Right
  C1 : PMIOPort  Port=5  Side=Left
  c : PMIOPort  Port=6  Side=Right
  A2 : PMIOPort  Port=7  Side=Left
  B2 : PMIOPort  Port=8  Side=Left
  C2 : PMIOPort  Port=9  Side=Left
  wires:
  gate/1 -> Ideal Switch1/1, Ideal Switch2/1, Ideal Switch3/1, Logical Operator/1
  Logical Operator/1 -> Ideal Switch4/1, Ideal Switch5/1, Ideal Switch6/1
  connections:
  A1/RConn1 -- Ideal Switch1/LConn1
  Ideal Switch1/RConn1 -- a/RConn1 -- Ideal Switch4/RConn1
  B1/RConn1 -- Ideal Switch2/LConn1
  Ideal Switch2/RConn1 -- Ideal Switch5/RConn1 -- b/RConn1
  C1/RConn1 -- Ideal Switch3/LConn1
  Ideal Switch3/RConn1 -- Ideal Switch6/RConn1 -- c/RConn1
  A2/RConn1 -- Ideal Switch4/LConn1
  B2/RConn1 -- Ideal Switch5/LConn1
  C2/RConn1 -- Ideal Switch6/LConn1

== system Test_FourMotor_PID_Ave/Detailed/Synchronous Motor & Drive4/Three-phase Inverter/Id computation ==
  m : Inport
  Vdc : Inport  Port=2
  Demux : Subsystem
  Demux1 : Subsystem
  Gain : Gain  Gain=Ron
  Math Function : Math  Operator=magnitude^2  SignedPower=on
  Math Function1 : Math  Operator=magnitude^2  SignedPower=on
  Math Function2 : Math  Operator=magnitude^2  SignedPower=on
  Product1 : Product  Inputs=*/  SaturateOnIntegerOverflow=on  OutDataTypeStr=Inherit: Same as first input
  Sum1 : Sum  Inputs=+++  SaturateOnIntegerOverflow=on
  Sum2 : Sum  Inputs=|++  SaturateOnIntegerOverflow=on
  Sum3 : Sum  SaturateOnIntegerOverflow=on
  Unit Delay1 : UnitDelay  SampleTime=Ts  HasFrameUpgradeWarning=on
  Unit Delay4 : UnitDelay  InitialCondition=1  SampleTime=Ts  HasFrameUpgradeWarning=on
  Vac x Ia : Product  SaturateOnIntegerOverflow=on  OutDataTypeStr=Inherit: Same as first input
  Vbc x Ib : Product  SaturateOnIntegerOverflow=on  OutDataTypeStr=Inherit: Same as first input
  Zero avoider : Saturate  UpperLimit=inf  LowerLimit=1
  Id : Outport  VectorParamsAs1DForOutWhenUnconnected=off
  wires:
  Sum2/1 -> Unit Delay1/1
  Sum3/1 -> Sum2/1
  Sum1/1 -> Gain/1
  Math Function2/1 -> Sum1/3
  Math Function/1 -> Sum1/1
  Math Function1/1 -> Sum1/2
  Demux1/3(Ic) -> Math Function2/1
  Demux1/2(Ib) -> Math Function1/1
  Demux1/1(Ia) -> Math Function/1
  Unit Delay4/1 -> Zero avoider/1
  Unit Delay1/1 -> Product1/1
  m/1 -> Demux1/1(m), Demux/1(m)
  Vac x Ia/1 -> Sum3/1
  Vbc x Ib/1 -> Sum3/2
  Vdc/1 -> Unit Delay4/1
  Demux/1(Vac) -> Vac x Ia/1
  Demux/2(Ia) -> Vac x Ia/2
  Demux/4(Ib) -> Vbc x Ib/2
  Demux/3(Vbc) -> Vbc x Ib/1
  Gain/1 -> Sum2/2
  Product1/1 -> Id/1
  Zero avoider/1 -> Product1/2

== system Test_FourMotor_PID_Ave/Detailed/Synchronous Motor & Drive4/Three-phase Inverter/Limit detection ==
  note: Limit = 1 saturation mode (voltage mode)
      | Limit = 0 normal mode (current mode)
  note: Low pass filter
  note: Low pass filter
  Vcc : Inport
  ctrl : Inport  Port=2
  Bus Selector1 : BusSelector  OutputSignals=m.Stator current is_d (A),m.Stator current is_q (A),m.Rotor speed wm (rad/s)  OutputAsBus=on
  Discrete Transfer Fcn1 : DiscreteTransferFcn  Numerator=[1-exp(-Ts*Fcs*2*pi)]  Denominator=[1 -exp(-Ts*Fcs*2*pi)]  SampleTime=Ts
  Discrete Transfer Fcn3 : DiscreteTransferFcn  Numerator=[1-exp(-Ts*Fcs*2*pi)]  Denominator=[1 -exp(-Ts*Fcs*2*pi)]  SampleTime=Ts
  Gain1 : Gain  Gain=0.9  SaturateOnIntegerOverflow=on  OutDataTypeStr=Inherit: Same as input  ParamDataTypeStr=Inherit: Same as input
  "Internal Vcc " : Fcn  Expr=pi/2*sqrt((Resistance*u(1)-Lq*p*u(3)*u(2))^2+(Resistance*u(2)+Ld*p*u(3)*u(1)+Flux*p*u(3))^2)
  Relational Operator : RelationalOperator  Operator=>  OutDataTypeStr=boolean  InputSameDT=off
  Relational Operator2 : RelationalOperator  Operator=<  OutDataTypeStr=boolean  InputSameDT=off
  S-R Flip-Flop : simulink_extras/Flip Flops/S-R Flip-Flop  initial_condition=0
  Terminator : Terminator
  Limit : Outport  VectorParamsAs1DForOutWhenUnconnected=off
  wires:
  Vcc/1 -> Discrete Transfer Fcn3/1
  Relational Operator/1 -> S-R Flip-Flop/1
  Relational Operator2/1 -> S-R Flip-Flop/2
  S-R Flip-Flop/1 -> Limit/1
  ctrl/1 -> Bus Selector1/1
  Bus Selector1/1 -> "Internal Vcc "/1
  "Internal Vcc "/1 -> Discrete Transfer Fcn1/1
  Discrete Transfer Fcn1/1 -> Relational Operator/1, Relational Operator2/1
  Gain1/1 -> Relational Operator2/2
  Discrete Transfer Fcn3/1 -> Gain1/1, Relational Operator/2
  S-R Flip-Flop/2 -> Terminator/1

== system Test_FourMotor_PID_Ave/Detailed/Synchronous Motor & Drive4/Three-phase Inverter/Output Resistance correction ==
  note: Vabc
  ctrl : Inport
  1/R : Gain  Gain=1/(100*Resistance)  SaturateOnIntegerOverflow=on  OutDataTypeStr=Inherit: Same as input  ParamDataTypeStr=Inherit: Same as input
  Bus Selector1 : BusSelector  OutputSignals=m.Stator voltage Vs_d (V),m.Stator voltage Vs_q (V),m.Rotor angle thetam (rad)
  Constant : Constant  Value=0
  Discrete Transfer Fcn1 : DiscreteTransferFcn  Numerator=[1-exp(-Ts/.001)]  Denominator=[1 -exp(-Ts/.001)]  SampleTime=Ts
  Discrete Transfer Fcn2 : DiscreteTransferFcn  Numerator=[1-exp(-Ts/.001)]  Denominator=[1 -exp(-Ts/.001)]  SampleTime=Ts
  Fcn : Fcn  Expr=sin(u)
  Fcn1 : Fcn  Expr=cos(u)
  Mux4 : Mux  Inputs=3
  Mux5 : Mux  Inputs=2
  dq0_to_abc Transformation : powerlib_extras/Measurements/dq0_to_abc Transformation
  poles : Gain  Gain=p  SaturateOnIntegerOverflow=on  OutDataTypeStr=Inherit: Same as input  ParamDataTypeStr=Inherit: Same as input
  "Iabc_r " : Outport  VectorParamsAs1DForOutWhenUnconnected=off
  wires:
  1/R/1 -> "Iabc_r "/1
  Bus Selector1/2 -> Discrete Transfer Fcn2/1  "<Stator voltage Vs_q (V)>"
  Bus Selector1/1 -> Discrete Transfer Fcn1/1  "<Stator voltage Vs_d (V)>"
  ctrl/1 -> Bus Selector1/1
  Mux4/1 -> dq0_to_abc Transformation/1
  Fcn/1 -> Mux5/1
  Fcn1/1 -> Mux5/2
  Mux5/1 -> dq0_to_abc Transformation/2
  Constant/1 -> Mux4/3
  dq0_to_abc Transformation/1 -> 1/R/1
  Discrete Transfer Fcn2/1 -> Mux4/2
  Discrete Transfer Fcn1/1 -> Mux4/1
  Bus Selector1/3 -> poles/1  "<Rotor angle thetam (rad)>"
  poles/1 -> Fcn/1, Fcn1/1

== system Test_FourMotor_PID_Ave/Detailed/Synchronous Motor & Drive4/VECT controller/Current Regulator ==
  Iabc* : Inport
  Iabc : Inport  Port=2
  Demux1 : Demux  Outputs=3
      settings: DisplayOption=none
  Demux2 : Demux  Outputs=3
      settings: DisplayOption=none
  Mux1 : Mux  Inputs=2
  Relay : Relay  OnSwitchValue=0  OffSwitchValue=0
  Relay1 : Relay  OnSwitchValue=0  OffSwitchValue=0
  Relay2 : Relay  OnSwitchValue=0  OffSwitchValue=0
  Sum : Sum  Inputs=-+  InputSameDT=on  SaturateOnIntegerOverflow=on  OutDataTypeStr=Inherit: Same as first input
  Sum1 : Sum  Inputs=-+  InputSameDT=on  SaturateOnIntegerOverflow=on  OutDataTypeStr=Inherit: Same as first input
  Sum2 : Sum  Inputs=-+  InputSameDT=on  SaturateOnIntegerOverflow=on  OutDataTypeStr=Inherit: Same as first input
  Sum3 : Sum  Inputs=+-
  Sum4 : Sum  Inputs=+-
  Pulses : Outport  InitialOutput=0  VectorParamsAs1DForOutWhenUnconnected=off
  wires:
  Sum/1 -> Relay/1
  Sum1/1 -> Relay1/1
  Demux1/1 -> Sum/1
  Demux1/2 -> Sum1/1
  Mux1/1 -> Pulses/1
  Iabc/1 -> Demux1/1
  Sum2/1 -> Relay2/1
  Demux1/3 -> Sum2/1
  Demux2/3 -> Sum2/2
  Demux2/2 -> Sum1/2
  Demux2/1 -> Sum/2
  Iabc*/1 -> Demux2/1
  Relay/1 -> Sum3/1
  Relay1/1 -> Sum3/2, Sum4/1
  Relay2/1 -> Sum4/2
  Sum3/1 -> Mux1/1
  Sum4/1 -> Mux1/2

== system Test_FourMotor_PID_Ave/Detailed/Synchronous Motor & Drive4/VECT controller/DQ-ABC ==
  "Iq* " : Inport
  "Id* " : Inport  Port=2
  Teta : Inport  Port=3
  Fcn : Fcn  Expr=sin(u)
  Fcn1 : Fcn  Expr=cos(u)
  Gain2 : Gain  SaturateOnIntegerOverflow=on  OutDataTypeStr=Inherit: Same as input  ParamDataTypeStr=Inherit: Same as input
  Gain3 : Gain  SaturateOnIntegerOverflow=on  OutDataTypeStr=Inherit: Same as input  ParamDataTypeStr=Inherit: Same as input
  Gain4 : Gain  SaturateOnIntegerOverflow=on  OutDataTypeStr=Inherit: Same as input  ParamDataTypeStr=Inherit: Same as input
  Mux : Mux
  Mux2 : Mux  Inputs=3
  ia : Fcn  Expr=-u[3]*u[2] + u[4]*u[1]
  ib : Fcn  Expr=(-u[1]+1.7320508*u[2])*u[4]*0.5+(u[2]+1.7320508*u[1])*u[3]*0.5
  ic : Sum  Inputs=--  InputSameDT=on  SaturateOnIntegerOverflow=on  OutDataTypeStr=Inherit: Same as first input
  Iabc* : Outport  InitialOutput=0  VectorParamsAs1DForOutWhenUnconnected=off
  wires:
  Fcn/1 -> Mux/2
  Fcn1/1 -> Mux/1
  Mux2/1 -> Iabc*/1
  Mux/1 -> ib/1, ia/1
  Teta/1 -> Fcn1/1, Fcn/1
  "Id* "/1 -> Mux/3
  "Iq* "/1 -> Mux/4
  Gain3/1 -> Mux2/2
  ic/1 -> Gain4/1
  Gain4/1 -> Mux2/3
  Gain2/1 -> Mux2/1
  ia/1 -> Gain2/1, ic/2
  ib/1 -> Gain3/1, ic/1

== system Test_FourMotor_PID_Ave/Detailed/Synchronous Motor & Drive4/VECT controller/Zero crossing detector ==
  En : Inport
  Iabc* : Inport  Port=2
  D Latch : simulink_extras/Flip Flops/D Latch
  D Latch1 : simulink_extras/Flip Flops/D Latch
  D Latch2 : simulink_extras/Flip Flops/D Latch
  Data Type Conversion : DataTypeConversion  SaturateOnIntegerOverflow=off  RndMeth=Floor
  Data Type Conversion2 : DataTypeConversion  SaturateOnIntegerOverflow=off  RndMeth=Floor
  Demux : Demux  Outputs=3
  Hit Crossing : HitCross
  Mux : Mux  Inputs=3
  Terminator : Terminator
  Terminator1 : Terminator
  Terminator2 : Terminator
  Enable : Outport  VectorParamsAs1DForOutWhenUnconnected=off
  wires:
  Data Type Conversion/1 -> D Latch/1, D Latch1/1, D Latch2/1
  Hit Crossing/1 -> Demux/1
  Demux/2 -> D Latch1/2
  Demux/3 -> D Latch2/2
  D Latch/1 -> Mux/1
  D Latch1/1 -> Mux/2
  D Latch2/1 -> Mux/3
  Mux/1 -> Data Type Conversion2/1
  Demux/1 -> D Latch/2
  En/1 -> Data Type Conversion/1
  Iabc*/1 -> Hit Crossing/1
  Data Type Conversion2/1 -> Enable/1
  D Latch/2 -> Terminator/1
  D Latch1/2 -> Terminator1/1
  D Latch2/2 -> Terminator2/1

== system Test_FourMotor_PID_Ave/Detailed/DC//DC Converter/PWM/Thermal Model/Subsystem ==
  IBus : Inport
  PToHeat : Gain  Gain=HEV_Param.DCDCConv.EPower2Heat  SaturateOnIntegerOverflow=on  OutDataTypeStr=Inherit: Same as input  ParamDataTypeStr=Inherit: Same as input
  Product : Product  RndMeth=Zero
  RLoss : Gain  Gain=HEV_Param.DCDCConv.Resistance_Losses  SaturateOnIntegerOverflow=on  OutDataTypeStr=Inherit: Same as input  ParamDataTypeStr=Inherit: Same as input
  Heat Flow : Outport  VectorParamsAs1DForOutWhenUnconnected=off
  wires:
  Product/1 -> RLoss/1
  IBus/1 -> Product/1, Product/2
  RLoss/1 -> PToHeat/1
  PToHeat/1 -> Heat Flow/1

== system Test_FourMotor_PID_Ave/Detailed/Synchronous Motor & Drive1/Three-phase Inverter/Id computation/Demux ==
  m : Inport
  Demux1 : Demux  Outputs=5
      settings: DisplayOption=none
  Terminator : Terminator
  Vac : Outport  VectorParamsAs1DForOutWhenUnconnected=off
  Ia : Outport  Port=2  VectorParamsAs1DForOutWhenUnconnected=off
  Vbc : Outport  Port=3  VectorParamsAs1DForOutWhenUnconnected=off
  Ib : Outport  Port=4  VectorParamsAs1DForOutWhenUnconnected=off
  wires:
  m/1 -> Demux1/1
  Demux1/5 -> Vbc/1  "Vbc"
  Demux1/4 -> Vac/1  "Vac"
  Demux1/2 -> Ib/1  "Ib"
  Demux1/1 -> Ia/1  "Ia"
  Demux1/3 -> Terminator/1  "Ic"

== system Test_FourMotor_PID_Ave/Detailed/Synchronous Motor & Drive1/Three-phase Inverter/Id computation/Demux1 ==
  m : Inport
  Demux1 : Demux  Outputs=5
      settings: DisplayOption=none
  Terminator1 : Terminator
  Terminator2 : Terminator
  Ia : Outport  VectorParamsAs1DForOutWhenUnconnected=off
  Ib : Outport  Port=2  VectorParamsAs1DForOutWhenUnconnected=off
  Ic : Outport  Port=3  VectorParamsAs1DForOutWhenUnconnected=off
  wires:
  Demux1/3 -> Ic/1  "Ic"
  Demux1/1 -> Ia/1  "Ia"
  Demux1/2 -> Ib/1  "Ib"
  Demux1/4 -> Terminator1/1  "Vac"
  Demux1/5 -> Terminator2/1  "Vbc"
  m/1 -> Demux1/1

== system Test_FourMotor_PID_Ave/Detailed/Synchronous Motor & Drive2/Three-phase Inverter/Id computation/Demux ==
  m : Inport
  Demux1 : Demux  Outputs=5
      settings: DisplayOption=none
  Terminator : Terminator
  Vac : Outport  VectorParamsAs1DForOutWhenUnconnected=off
  Ia : Outport  Port=2  VectorParamsAs1DForOutWhenUnconnected=off
  Vbc : Outport  Port=3  VectorParamsAs1DForOutWhenUnconnected=off
  Ib : Outport  Port=4  VectorParamsAs1DForOutWhenUnconnected=off
  wires:
  m/1 -> Demux1/1
  Demux1/5 -> Vbc/1  "Vbc"
  Demux1/4 -> Vac/1  "Vac"
  Demux1/2 -> Ib/1  "Ib"
  Demux1/1 -> Ia/1  "Ia"
  Demux1/3 -> Terminator/1  "Ic"

== system Test_FourMotor_PID_Ave/Detailed/Synchronous Motor & Drive2/Three-phase Inverter/Id computation/Demux1 ==
  m : Inport
  Demux1 : Demux  Outputs=5
      settings: DisplayOption=none
  Terminator1 : Terminator
  Terminator2 : Terminator
  Ia : Outport  VectorParamsAs1DForOutWhenUnconnected=off
  Ib : Outport  Port=2  VectorParamsAs1DForOutWhenUnconnected=off
  Ic : Outport  Port=3  VectorParamsAs1DForOutWhenUnconnected=off
  wires:
  Demux1/3 -> Ic/1  "Ic"
  Demux1/1 -> Ia/1  "Ia"
  Demux1/2 -> Ib/1  "Ib"
  Demux1/4 -> Terminator1/1  "Vac"
  Demux1/5 -> Terminator2/1  "Vbc"
  m/1 -> Demux1/1

== system Test_FourMotor_PID_Ave/Detailed/Synchronous Motor & Drive3/Three-phase Inverter/Id computation/Demux ==
  m : Inport
  Demux1 : Demux  Outputs=5
      settings: DisplayOption=none
  Terminator : Terminator
  Vac : Outport  VectorParamsAs1DForOutWhenUnconnected=off
  Ia : Outport  Port=2  VectorParamsAs1DForOutWhenUnconnected=off
  Vbc : Outport  Port=3  VectorParamsAs1DForOutWhenUnconnected=off
  Ib : Outport  Port=4  VectorParamsAs1DForOutWhenUnconnected=off
  wires:
  m/1 -> Demux1/1
  Demux1/5 -> Vbc/1  "Vbc"
  Demux1/4 -> Vac/1  "Vac"
  Demux1/2 -> Ib/1  "Ib"
  Demux1/1 -> Ia/1  "Ia"
  Demux1/3 -> Terminator/1  "Ic"

== system Test_FourMotor_PID_Ave/Detailed/Synchronous Motor & Drive3/Three-phase Inverter/Id computation/Demux1 ==
  m : Inport
  Demux1 : Demux  Outputs=5
      settings: DisplayOption=none
  Terminator1 : Terminator
  Terminator2 : Terminator
  Ia : Outport  VectorParamsAs1DForOutWhenUnconnected=off
  Ib : Outport  Port=2  VectorParamsAs1DForOutWhenUnconnected=off
  Ic : Outport  Port=3  VectorParamsAs1DForOutWhenUnconnected=off
  wires:
  Demux1/3 -> Ic/1  "Ic"
  Demux1/1 -> Ia/1  "Ia"
  Demux1/2 -> Ib/1  "Ib"
  Demux1/4 -> Terminator1/1  "Vac"
  Demux1/5 -> Terminator2/1  "Vbc"
  m/1 -> Demux1/1

== system Test_FourMotor_PID_Ave/Detailed/Synchronous Motor & Drive4/Three-phase Inverter/Id computation/Demux ==
  m : Inport
  Demux1 : Demux  Outputs=5
      settings: DisplayOption=none
  Terminator : Terminator
  Vac : Outport  VectorParamsAs1DForOutWhenUnconnected=off
  Ia : Outport  Port=2  VectorParamsAs1DForOutWhenUnconnected=off
  Vbc : Outport  Port=3  VectorParamsAs1DForOutWhenUnconnected=off
  Ib : Outport  Port=4  VectorParamsAs1DForOutWhenUnconnected=off
  wires:
  m/1 -> Demux1/1
  Demux1/5 -> Vbc/1  "Vbc"
  Demux1/4 -> Vac/1  "Vac"
  Demux1/2 -> Ib/1  "Ib"
  Demux1/1 -> Ia/1  "Ia"
  Demux1/3 -> Terminator/1  "Ic"

== system Test_FourMotor_PID_Ave/Detailed/Synchronous Motor & Drive4/Three-phase Inverter/Id computation/Demux1 ==
  m : Inport
  Demux1 : Demux  Outputs=5
      settings: DisplayOption=none
  Terminator1 : Terminator
  Terminator2 : Terminator
  Ia : Outport  VectorParamsAs1DForOutWhenUnconnected=off
  Ib : Outport  Port=2  VectorParamsAs1DForOutWhenUnconnected=off
  Ic : Outport  Port=3  VectorParamsAs1DForOutWhenUnconnected=off
  wires:
  Demux1/3 -> Ic/1  "Ic"
  Demux1/1 -> Ia/1  "Ia"
  Demux1/2 -> Ib/1  "Ib"
  Demux1/4 -> Terminator1/1  "Vac"
  Demux1/5 -> Terminator2/1  "Vbc"
  m/1 -> Demux1/1

== matlab function Test_FourMotor_PID_Ave/Detailed/Synchronous Motor & Drive3/VECT controller/Embedded MATLAB Function1 ==
  data: iqn_opt input; Ten input; iqn output; w input; Vdc input; params input; idn output
function [iqn,idn] = fcn(iqn_opt,Ten,w,Vdc,params)
% This block supports the Embedded MATLAB subset.
% See the help menu for details.

kFact = 0.9;
Ld = params(1);
Lq = params(2);
lam = params(3);
p = params(4);
ib = params(5);
Vs = Vdc/(pi/2)*kFact;
ten = abs(Ten);
iqn = sign(Ten)*iqn_opt;
if Ten == 0 && w == 0
    idn = 0;
elseif iqn == 0
    idn = -(lam*p*w-Vs*kFact)/(p*Ld*w*ib);
else
    idn = 1-Ten/iqn;
end
if sqrt((-Lq*p*w*iqn*ib)^2+(Ld*p*w*idn*ib+lam*p*w)^2) >= Vs 
    vs = Vs;
    k1 = 2*lam*Ld/(ib*Lq^2);
    k2 = Ld^2/Lq^2;
    k3 = lam^2/(ib^2*Lq^2)+k2;
    
    g2 = -vs^2/(p^2*ib^2*Lq^2*w^2) + k1 + k3;
    g3 = -k1*ten-2*ten*k2;
    g4 = k2*ten^2;
    
    a1 = abs(-768*g4^3+384*g4^2*g2^2-48*g4*g2^4-432*g2*g4*g3^2+81*g3^4+12*g3^2*g2^3)^(1/2);
    a2 = (-288*g2*g4+108*g3^2+8*g2^3+12*a1)^(1/3);
    a3 = (-4*g2+a2+48/a2*g4+4/a2*g2^2)^(1/2);
    iqn = (1/12*6^(1/2)*a3+1/12*abs(-48*g2-6*a2-288/a2*g4-24/a2*g2^2-72/a3*g3*6^(1/2))^(1/2));
    iqn = sign(Ten)*iqn;

    idn = 1-Ten/iqn;
end

== matlab function Test_FourMotor_PID_Ave/Detailed/Synchronous Motor & Drive1/VECT Controller/Embedded MATLAB Function1 ==
  data: iqn_opt input; Ten input; iqn output; w input; Vdc input; params input; idn output
function [iqn,idn] = fcn(iqn_opt,Ten,w,Vdc,params)
% This block supports the Embedded MATLAB subset.
% See the help menu for details.

kFact = 0.9;
Ld = params(1);
Lq = params(2);
lam = params(3);
p = params(4);
ib = params(5);
Vs = Vdc/(pi/2)*kFact;
ten = abs(Ten);
iqn = sign(Ten)*iqn_opt;
if Ten == 0 && w == 0
    idn = 0;
elseif iqn == 0
    idn = -(lam*p*w-Vs*kFact)/(p*Ld*w*ib);
else
    idn = 1-Ten/iqn;
end
if sqrt((-Lq*p*w*iqn*ib)^2+(Ld*p*w*idn*ib+lam*p*w)^2) >= Vs 
    vs = Vs;
    k1 = 2*lam*Ld/(ib*Lq^2);
    k2 = Ld^2/Lq^2;
    k3 = lam^2/(ib^2*Lq^2)+k2;
    
    g2 = -vs^2/(p^2*ib^2*Lq^2*w^2) + k1 + k3;
    g3 = -k1*ten-2*ten*k2;
    g4 = k2*ten^2;
    
    a1 = abs(-768*g4^3+384*g4^2*g2^2-48*g4*g2^4-432*g2*g4*g3^2+81*g3^4+12*g3^2*g2^3)^(1/2);
    a2 = (-288*g2*g4+108*g3^2+8*g2^3+12*a1)^(1/3);
    a3 = (-4*g2+a2+48/a2*g4+4/a2*g2^2)^(1/2);
    iqn = (1/12*6^(1/2)*a3+1/12*abs(-48*g2-6*a2-288/a2*g4-24/a2*g2^2-72/a3*g3*6^(1/2))^(1/2));
    iqn = sign(Ten)*iqn;

    idn = 1-Ten/iqn;
end
